simulink model "MEEN5210_HW8_Prob2"  (R2017a)
settings: Solver=VariableStepAuto  StartTime=0.0  StopTime=10.0  RelTol=1e-3
values from neighbouring files (symbols this model uses):
  A = [[-3 5];[0 -2]]    [MEEN5210_HW8_ControlsAndObservers.m]
  B = [1 -1].'    [MEEN5210_HW8_ControlsAndObservers.m]
  C = [1 0]    [MEEN5210_HW8_ControlsAndObservers.m]
  D = [0]    [MEEN5210_HW8_ControlsAndObservers.m]
  L = double(linsolve(meatMat, potatoesMat))    [MEEN5210_HW8_ControlsAndObservers.m]
  x0 = [0 0].'    [MEEN5210_HW8_ControlsAndObservers.m]
settings Model: Creator=jfrancis  LastModifiedBy=jfrancis

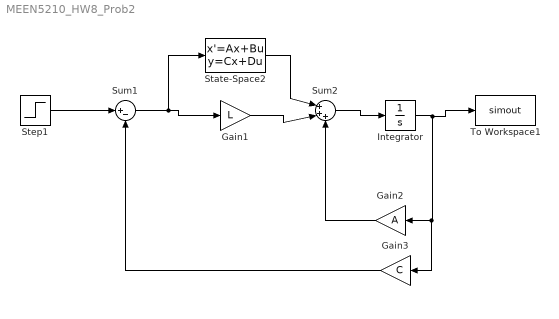
== system MEEN5210_HW8_Prob2 ==
  Gain1 : Gain  Gain=L
  Gain2 : Gain  Gain=A
  Gain3 : Gain  Gain=C
  Integrator : Integrator
  State-Space2 : StateSpace  A=A  B=B  C=C  D=D  X0=x0
  Step1 : Step  SampleTime=0
  Sum1 : Sum  Inputs=|+-
  Sum2 : Sum  Inputs=|+++
  To Workspace1 : ToWorkspace  VariableName=simout  SaveFormat=Timeseries  SampleTime=-1
  wires:
  Integrator/1 -> To Workspace1/1, Gain3/1, Gain2/1
  Gain2/1 -> Sum2/3
  Gain3/1 -> Sum1/2
  Sum1/1 -> State-Space2/1, Gain1/1
  Gain1/1 -> Sum2/2
  Sum2/1 -> Integrator/1
  Step1/1 -> Sum1/1
  State-Space2/1 -> Sum2/1
